simulink model "aerosonde_controlled"  (Simulink 7.7)
settings: Solver=ode3  StartTime=0.0  StopTime=200  FixedStep=20e-3  RelTol=1e-6
values from neighbouring files (symbols this model uses):
  aerosonde = aerosonde_data    [aerosonde_initialize.m]    (also in aerosonde_trimlin.m)
  chi_trim = 0    [aerosonde_initialize.m]
  eta_trim = -0.1    [aerosonde_initialize.m]
  euler_0 = [theta_trim; 0; 0]    [aerosonde_initialize.m]    (also in aerosonde_trimlin.m = xtrim(11:13))
  flap = 0    [aerosonde_initialize.m]
  fuel_0 = 2    [aerosonde_initialize.m]    (also in aerosonde_trimlin.m = xtrim(10))
  h_trim = 500    [aerosonde_initialize.m]
  ignition = 1    [aerosonde_initialize.m]
  Kari = 0.5    [aerosonde_initialize.m]
  Kd_Ye = 0.6    [aerosonde_initialize.m]
  Kd_Ze = -0.05    [aerosonde_initialize.m]
  Ki_phi = -0.1    [aerosonde_initialize.m]
  Ki_psi = 0.001    [aerosonde_initialize.m]
  Ki_theta = -0.8    [aerosonde_initialize.m]
  Ki_u = 0.15    [aerosonde_initialize.m]
  Ki_Ye = 0.0025    [aerosonde_initialize.m]
  Ki_Ze = -0.0001    [aerosonde_initialize.m]
  Kp_phi = -0.2    [aerosonde_initialize.m]
  Kp_psi = 0.7    [aerosonde_initialize.m]
  Kp_theta = -0.8    [aerosonde_initialize.m]
  Kp_u = 0.5    [aerosonde_initialize.m]
  Kp_Xe = 0.125    [aerosonde_initialize.m]
  Kp_Ye = 0.18    [aerosonde_initialize.m]
  Kp_Ze = -0.03    [aerosonde_initialize.m]
  Kphi_xi = -0.2    [aerosonde_initialize.m]
  Kq_eta = -0.28    [aerosonde_initialize.m]
  Kr_zeta = -0.25    [aerosonde_initialize.m]
  Ktheta_eta = -1    [aerosonde_initialize.m]
  latitude = 52.073105    [aerosonde_initialize.m]
  longitude = -000.616697    (= -0.616697)    [aerosonde_initialize.m]
  mixture = 13    [aerosonde_initialize.m]
  Omega_0 = 5000*pi/30    (= 523.598775598)    [aerosonde_initialize.m]    (also in aerosonde_trimlin.m = xtrim(14))
  position_0 = [0; 0; -h_trim]    [aerosonde_initialize.m]
  q_trim = 0    [aerosonde_initialize.m]
  rates_0 = [0; q_trim ; 0]    [aerosonde_initialize.m]    (also in aerosonde_trimlin.m = xtrim(7:9))
  tau_trim = 0.4    [aerosonde_initialize.m]
  theta_trim = 0    [aerosonde_initialize.m]
  Tr = 0.75    [aerosonde_initialize.m]
  Ue_VL = 25    [aerosonde_initialize.m]
  Ve_VL = 0    [aerosonde_initialize.m]
  velocity_0 = [23; 0; 0]    [aerosonde_initialize.m]    (also in aerosonde_trimlin.m = xtrim(1:3))
  We_VL = 0    [aerosonde_initialize.m]
  Xe0_VL = position_0(1)    [aerosonde_initialize.m]
  xi_trim = 0    [aerosonde_initialize.m]
  Ye0_VL = position_0(2)    [aerosonde_initialize.m]
  Ze0_VL = position_0(3)    [aerosonde_initialize.m]
  zeta_trim = 0    [aerosonde_initialize.m]
undefined symbols (not defined in the file or in its folder): Earth, F, m, MIL, rad, s, WGS84
libraries: aerolibasang x4, aerolibbdyn x3, aerolibfltsims x3, simulink_extras x3, aerolibwind2 x3, aerolibtransform2 x2, aerolibatmos2 x2, aerolibconvert2 x2, simulink x2, aerolibadyn x1, aerolib6dof2 x1, aerolibutil x1
(part 2 of 2)

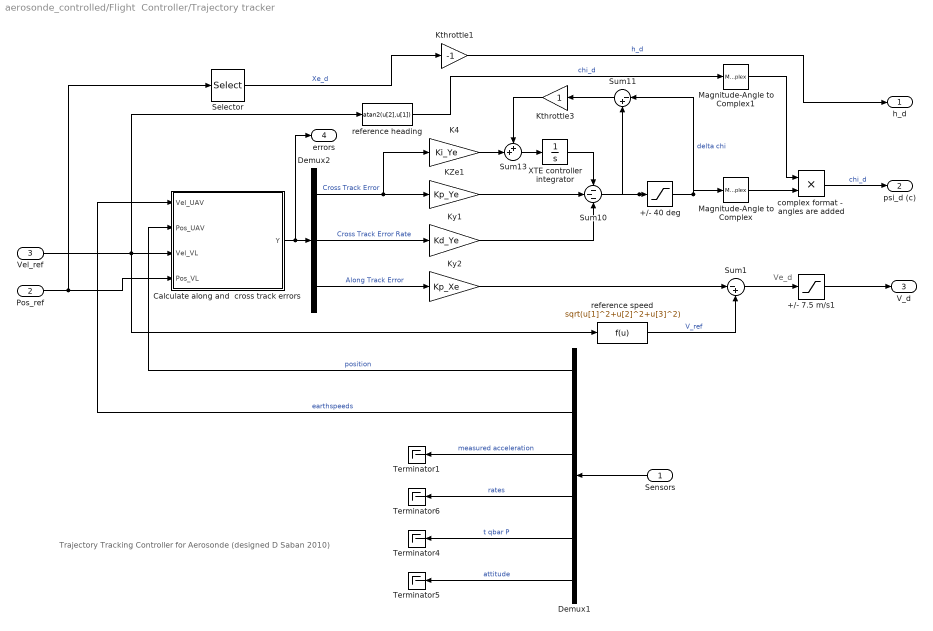
== system aerosonde_controlled/Flight  Controller/Trajectory tracker ==
  note: Ve_d
  note: Trajectory Tracking Controller
      | for Aerosonde
      | (designed D Saban 2010)
  Sensors : Inport  PortDimensions=18
  Pos_ref : Inport  Port=2
  Vel_ref : Inport  Port=3
  +/- 40 deg : Saturate  UpperLimit=+40.0*pi/180  LowerLimit=-40*pi/180  ZeroCross=off
  +/- 7.5 m/s1 : Saturate  UpperLimit=90  LowerLimit=18  ZeroCross=off
  Calculate along and  cross track errors : Stateflow chart  TreatAsAtomicUnit=on
  Demux1 : Demux  Outputs=[3 3 3 3 3 3]
  Demux2 : Demux  Outputs=3
  K4 : Gain  Gain=Ki_Ye
  KZe1 : Gain  Gain=Kp_Ye
  Kthrottle1 : Gain  Gain=-1
  Kthrottle3 : Gain
  Ky1 : Gain  Gain=Kd_Ye
  Ky2 : Gain  Gain=Kp_Xe
  Magnitude-Angle to Complex : MagnitudeAngleToComplex  Input=Angle  ConstantPart=1
  Magnitude-Angle to Complex1 : MagnitudeAngleToComplex  Input=Angle  ConstantPart=1
  Selector : Selector  InputPortWidth=3  IndexOptions=Index vector (dialog)  Indices=3  OutputSizes=1
  Sum1 : Sum  Inputs=|-+
  Sum10 : Sum  Inputs=---
  Sum11 : Sum  Inputs=|-+
  Sum13 : Sum  Inputs=++|
  Terminator{1,4..6} (4 alike) : Terminator
  XTE controller integrator : Integrator
  complex format -  angles are added : Product  RndMeth=Zero
  reference heading : Fcn  Expr=atan2(u[2],u[1])
  reference speed : Fcn  Expr=sqrt(u[1]^2+u[2]^2+u[3]^2)
  h_d : Outport
  psi_d (c) : Outport  Port=2
  V_d : Outport  Port=3
  errors : Outport  Port=4
  wires:
  KZe1/1 -> Sum10/2
  K4/1 -> Sum13/2
  Sum13/1 -> XTE controller integrator/1
  XTE controller integrator/1 -> Sum10/1
  Sum10/1 -> Sum11/2, +/- 40 deg/1
  Sum11/1 -> Kthrottle3/1
  Kthrottle3/1 -> Sum13/1
  Ky1/1 -> Sum10/3
  Demux2/1 -> KZe1/1, K4/1  "Cross Track Error"
  Calculate along and  cross track errors/1(Y) -> Demux2/1, errors/1
  Ky2/1 -> Sum1/1
  Pos_ref/1 -> Calculate along and  cross track errors/4(Pos_VL), Selector/1
  Vel_ref/1 -> Calculate along and  cross track errors/3(Vel_VL), reference speed/1, reference heading/1
  Demux2/3 -> Ky2/1  "Along Track Error"
  Demux2/2 -> Ky1/1  "Cross Track Error Rate"
  Demux1/2 -> Calculate along and  cross track errors/1(Vel_UAV)  "earthspeeds"
  Demux1/3 -> Terminator1/1  "measured acceleration"
  Sensors/1 -> Demux1/1
  Demux1/5 -> Terminator4/1  "t qbar P"
  Demux1/1 -> Calculate along and  cross track errors/2(Pos_UAV)  "position"
  Demux1/4 -> Terminator6/1  "rates"
  Demux1/6 -> Terminator5/1  "attitude"
  Selector/1 -> Kthrottle1/1  "Xe_d"
  Kthrottle1/1 -> h_d/1  "h_d"
  Sum1/1 -> +/- 7.5 m/s1/1
  reference speed/1 -> Sum1/2  "V_ref"
  +/- 7.5 m/s1/1 -> V_d/1
  complex format -  angles are added/1 -> psi_d (c)/1  "chi_d"
  +/- 40 deg/1 -> Sum11/1, Magnitude-Angle to Complex/1  "delta chi"
  reference heading/1 -> Magnitude-Angle to Complex1/1  "chi_d"
  Magnitude-Angle to Complex/1 -> complex format -  angles are added/2
  Magnitude-Angle to Complex1/1 -> complex format -  angles are added/1

== system aerosonde_controlled/FlightGear visualization/Flat Earth to LLA ==
  note: Flat Earth to LLA
  Xe : Inport
  altitude0 : Inport  Port=2
  Angle Conversion : aerolibconvert2/Angle Conversion  SystemSampleTime=-1  IU=deg  OU=rad
  Demux2 : Demux  Outputs=2
  Flat Earth to LLA : aerolibtransform2/Flat Earth to LLA  SystemSampleTime=-1  units=Metric (MKS)  ptype=Earth (WGS84)  F=1/298.257223563  R=6378137  LL0=[latitude longitude]  psi=0
  longitude l : Outport
  latitude mu : Outport  Port=2
  altitude h : Outport  Port=3
  wires:
  Flat Earth to LLA/1 -> Angle Conversion/1
  Demux2/1 -> latitude mu/1  "latitude"
  Demux2/2 -> longitude l/1
  Xe/1 -> Flat Earth to LLA/1
  altitude0/1 -> Flat Earth to LLA/2
  Flat Earth to LLA/2 -> altitude h/1  "altitude"
  Angle Conversion/1 -> Demux2/1

== system aerosonde_controlled/FlightGear visualization/phidot thetadot psidot ==
  pqr : Inport
  phi theta psi : Inport  Port=2
  Concatenate1 : Concatenate  NumInputs=3  Mode=Vector
  Concatenate2 : Concatenate  NumInputs=3  Mode=Vector
  SinCos : aerolibobsolete/SinCos  SystemSampleTime=-1
  keep angles  in range [-pi pi] : Trigonometry  Operator=atan2
  phidot : Fcn  Expr=u[1]+(u[2]*u[4]+u[3]*u[7])*(u[5]/u[8])
  psidot : Fcn  Expr=(u[2]*u[4]+u[3]*u[7])/u[8]
  thetadot : Fcn  Expr=u[2]*u[7]-u[3]*u[4]
  ptp_earth : Outport
  ptp_dot : Outport  Port=2
  wires:
  SinCos/2 -> Concatenate1/3, keep angles  in range [-pi pi]/2
  SinCos/1 -> Concatenate1/2, keep angles  in range [-pi pi]/1
  Concatenate2/1 -> ptp_dot/1
  phidot/1 -> Concatenate2/1
  thetadot/1 -> Concatenate2/2
  psidot/1 -> Concatenate2/3
  phi theta psi/1 -> SinCos/1
  pqr/1 -> Concatenate1/1
  Concatenate1/1 -> thetadot/1, phidot/1, psidot/1
  keep angles  in range [-pi pi]/1 -> ptp_earth/1

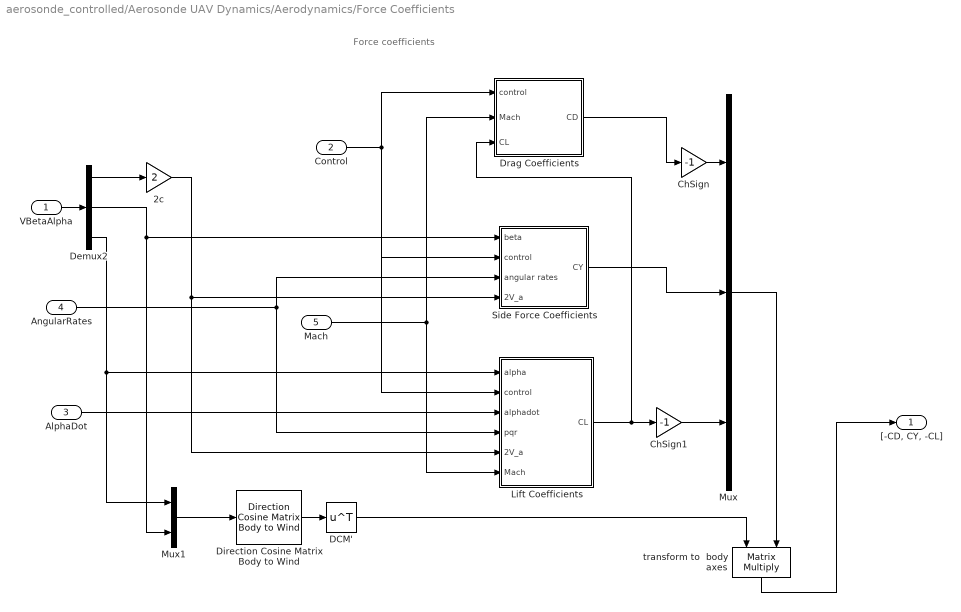
== system aerosonde_controlled/Aerosonde UAV Dynamics/Aerodynamics/Force Coefficients ==
  note: Force coefficients
  VBetaAlpha : Inport  PortDimensions=[3 1]
  Control : Inport  Port=2  PortDimensions=[4 1]
  AlphaDot : Inport  Port=3
  AngularRates : Inport  Port=4  PortDimensions=[3 1]
  Mach : Inport  Port=5  PortDimensions=1
  2c : Gain  Gain=2  SaturateOnIntegerOverflow=on  OutDataTypeStr=Inherit: Same as input  ParamDataTypeStr=Inherit: Same as input
  ChSign : Gain  Gain=-1  SaturateOnIntegerOverflow=on  OutDataTypeStr=Inherit: Same as input  ParamDataTypeStr=Inherit: Same as input
  ChSign1 : Gain  Gain=-1  SaturateOnIntegerOverflow=on  OutDataTypeStr=Inherit: Same as input  ParamDataTypeStr=Inherit: Same as input
  DCM' : Math  Operator=transpose  SaturateOnIntegerOverflow=on
  Demux2 : Demux  Outputs=3
  Direction Cosine Matrix Body to Wind : aerolibtransform2/Direction Cosine Matrix Body to Wind  SystemSampleTime=-1
  Drag Coefficients : Subsystem
  Lift Coefficients : Subsystem
  Mux : Mux  Inputs=3
  Mux1 : Mux  Inputs=2
  Side Force Coefficients : Subsystem
  transform to  body axes : Product  Inputs=**  Multiplication=Matrix(*)  SaturateOnIntegerOverflow=on  InputSameDT=on  OutDataTypeStr=Inherit: Same as first input
  "[-CD, CY, -CL]" : Outport
  wires:
  Mux1/1 -> Direction Cosine Matrix Body to Wind/1
  DCM'/1 -> transform to  body axes/1
  Mux/1 -> transform to  body axes/2
  Direction Cosine Matrix Body to Wind/1 -> DCM'/1
  transform to  body axes/1 -> "[-CD, CY, -CL]"/1
  Demux2/2 -> Mux1/2, Side Force Coefficients/1(beta)
  Demux2/1 -> 2c/1
  VBetaAlpha/1 -> Demux2/1
  ChSign1/1 -> Mux/3
  ChSign/1 -> Mux/1
  Side Force Coefficients/1(CY) -> Mux/2
  Drag Coefficients/1(CD) -> ChSign/1
  Lift Coefficients/1(CL) -> Drag Coefficients/3(CL), ChSign1/1
  Mach/1 -> Drag Coefficients/2(Mach), Lift Coefficients/6(Mach)
  AngularRates/1 -> Side Force Coefficients/3(angular rates), Lift Coefficients/4(pqr)
  AlphaDot/1 -> Lift Coefficients/3(alphadot)
  Control/1 -> Lift Coefficients/2(control), Side Force Coefficients/2(control), Drag Coefficients/1(control)
  Demux2/3 -> Lift Coefficients/1(alpha), Mux1/1
  2c/1 -> Side Force Coefficients/4(2V_a), Lift Coefficients/5(2V_a)

== system aerosonde_controlled/Aerosonde UAV Dynamics/Aerodynamics/Moment Coefficients ==
  note: Moment coefficients
  VBetaAlpha : Inport  PortDimensions=[3 1]
  Control : Inport  Port=2  PortDimensions=[4 1]
  AlphaDot : Inport  Port=3
  AngularRates : Inport  Port=4  PortDimensions=[3 1]
  Mach : Inport  Port=5  PortDimensions=1
  2c : Gain  Gain=2  SaturateOnIntegerOverflow=on  OutDataTypeStr=Inherit: Same as input  ParamDataTypeStr=Inherit: Same as input
  Demux1 : Demux  Outputs=3
  Mux : Mux  Inputs=3
  Pitch Moment Coefficients : Subsystem
  Roll Moment Coefficients : Subsystem
  Yaw Moment Coefficients : Subsystem
  "[-Cl, Cm, -Cn]" : Outport
  wires:
  Demux1/2 -> Yaw Moment Coefficients/1(beta), Roll Moment Coefficients/1(beta)
  Demux1/3 -> Pitch Moment Coefficients/1(alpha)
  Mach/1 -> Pitch Moment Coefficients/6(Mach)
  Yaw Moment Coefficients/1(Cn) -> Mux/3
  VBetaAlpha/1 -> Demux1/1
  2c/1 -> Pitch Moment Coefficients/5(2V_a), Yaw Moment Coefficients/4(2V_a), Roll Moment Coefficients/4(2V)
  Demux1/1 -> 2c/1
  Control/1 -> Roll Moment Coefficients/2(control), Yaw Moment Coefficients/2(control), Pitch Moment Coefficients/2(control)
  AlphaDot/1 -> Pitch Moment Coefficients/3(alphadot)
  AngularRates/1 -> Roll Moment Coefficients/3(angular rates), Yaw Moment Coefficients/3(angular rates), Pitch Moment Coefficients/4(pqr)
  Mux/1 -> "[-Cl, Cm, -Cn]"/1
  Pitch Moment Coefficients/1(Cm) -> Mux/2
  Roll Moment Coefficients/1(Cl) -> Mux/1

== system aerosonde_controlled/Aerosonde UAV Dynamics/Aerodynamics/Wind-axes Velocities ==
  VelB : Inport
  WindB : Inport  Port=2
  a : Inport  Port=3
  rho : Inport  Port=4
  VelBdot : Inport  Port=5
  Calculate  alphadot : Subsystem
  Derivative : Derivative
  Dynamic Pressure : aerolibasang/Dynamic Pressure  SystemSampleTime=-1
  "Incidence, Sideslip, & Airspeed" : aerolibasang/Incidence, Sideslip, & Airspeed  SystemSampleTime=-1
  Mach Number : aerolibasang/Mach Number  SystemSampleTime=-1
  Mux1 : Mux  Inputs=3
  Sum1 : Sum  Inputs=|+-  SaturateOnIntegerOverflow=on  InputSameDT=on  OutDataTypeStr=Inherit: Same as first input
  Sum2 : Sum  Inputs=-+|  SaturateOnIntegerOverflow=on  InputSameDT=on  OutDataTypeStr=Inherit: Same as first input
  VBetaAlpha : Outport
  Mach : Outport  Port=2
  qbar (pdyn) : Outport  Port=3
  alphadot : Outport  Port=4
  wires:
  Derivative/1 -> Sum2/1
  Sum2/1 -> Calculate  alphadot/1("[Udot Vdot Wdot]")
  VelBdot/1 -> Sum2/2
  Calculate  alphadot/1(alphadot) -> alphadot/1
  "Incidence, Sideslip, & Airspeed"/2 -> Mux1/2
  "Incidence, Sideslip, & Airspeed"/1 -> Mux1/3
  Dynamic Pressure/1 -> qbar (pdyn)/1
  rho/1 -> Dynamic Pressure/2
  a/1 -> Mach Number/2
  Mach Number/1 -> Mach/1
  WindB/1 -> Derivative/1, Sum1/2
  VelB/1 -> Sum1/1
  Mux1/1 -> VBetaAlpha/1
  "Incidence, Sideslip, & Airspeed"/3 -> Mux1/1
  Sum1/1 -> Calculate  alphadot/2("[U V W]"), Dynamic Pressure/1, Mach Number/1, "Incidence, Sideslip, & Airspeed"/1

== system aerosonde_controlled/Aerosonde UAV Dynamics/Propulsion System/Fixed-pitch Propeller ==
  note: Fixed-pitch
      | Propeller
  Airspeed : Inport  OutDataTypeStr=double  PortDimensions=1
  rho : Inport  Port=2  OutDataTypeStr=double  PortDimensions=1
  Omega : Inport  Port=3  OutDataTypeStr=double  PortDimensions=1
  4 R^4 / pi^2 : Gain  Gain=4*Rprop^4/pi^2  SaturateOnIntegerOverflow=on  OutDataTypeStr=Inherit: Same as input  ParamDataTypeStr=Inherit: Same as input
  4 R^5/ pi^3 : Gain  Gain=-4*Rprop^5/pi^3  SaturateOnIntegerOverflow=on  OutDataTypeStr=Inherit: Same as input  ParamDataTypeStr=Inherit: Same as input
  Coeff of Power : Lookup  InputValues=J  Table=CP  SaturateOnIntegerOverflow=on
  Coefficient  of Thrust : Lookup  InputValues=J  Table=CT  SaturateOnIntegerOverflow=on
  Omega^2 : Math  Operator=square  SaturateOnIntegerOverflow=on
  Va/Omega : Product  Inputs=*/  SaturateOnIntegerOverflow=on  InputSameDT=on  OutDataTypeStr=Inherit: Same as first input
  pi/R : Gain  Gain=pi/Rprop  SaturateOnIntegerOverflow=on  OutDataTypeStr=Inherit: Same as input  ParamDataTypeStr=Inherit: Same as input
  "rho Omega^2 " : Product  SaturateOnIntegerOverflow=on  InputSameDT=on  OutDataTypeStr=Inherit: Same as first input
  rho Omega^2 C_P : Product  SaturateOnIntegerOverflow=on  InputSameDT=on  OutDataTypeStr=Inherit: Same as first input
  rho Omega^2 C_T : Product  SaturateOnIntegerOverflow=on  InputSameDT=on  OutDataTypeStr=Inherit: Same as first input
  Fprop : Outport
  Mprop : Outport  Port=2
  wires:
  "rho Omega^2 "/1 -> rho Omega^2 C_P/2, rho Omega^2 C_T/2
  Omega^2/1 -> "rho Omega^2 "/1
  rho/1 -> "rho Omega^2 "/2
  4 R^5/ pi^3/1 -> Mprop/1  "torque"
  4 R^4 / pi^2/1 -> Fprop/1  "thrust"
  Airspeed/1 -> Va/Omega/1
  pi/R/1 -> Coeff of Power/1, Coefficient  of Thrust/1  "advance ratio"
  rho Omega^2 C_P/1 -> 4 R^5/ pi^3/1
  rho Omega^2 C_T/1 -> 4 R^4 / pi^2/1
  Coefficient  of Thrust/1 -> rho Omega^2 C_T/1
  Va/Omega/1 -> pi/R/1
  Omega/1 -> Va/Omega/2, Omega^2/1
  Coeff of Power/1 -> rho Omega^2 C_P/1

== system aerosonde_controlled/Aerosonde UAV Dynamics/Propulsion System/Piston Engine ==
  note: Compute MAP from
      | throttle area fraction
  note: Engine parameter
      | look-up tables
  Thr : Inport  OutDataTypeStr=double  PortDimensions=1
  Mix : Inport  Port=2  OutDataTypeStr=double  PortDimensions=1
  Omega : Inport  Port=3  OutDataTypeStr=double  PortDimensions=1
  P_atm : Inport  Port=4  OutDataTypeStr=double  PortDimensions=1
  T : Inport  Port=5  OutDataTypeStr=double  PortDimensions=1
  Altitude correction  for  Power : Subsystem
  Engine torque : Product  Inputs=*/  SaturateOnIntegerOverflow=on  InputSameDT=on  OutDataTypeStr=Inherit: Same as first input
  Fuel flow LUT : Lookup2D  RowIndex=RPM  ColumnIndex=MAP  Table=fflow  SaturateOnIntegerOverflow=on  InputSameDT=on
  Get air flow : Product  SaturateOnIntegerOverflow=on  InputSameDT=on  OutDataTypeStr=Inherit: Same as first input
  Intake : Subsystem
  Power LUT : Lookup2D  RowIndex=RPM  ColumnIndex=MAP  Table=Power  SaturateOnIntegerOverflow=on  InputSameDT=on
  Power at altitude : Product  SaturateOnIntegerOverflow=on  InputSameDT=on  OutDataTypeStr=Inherit: Same as first input
  g/hr 2 kg/s : Gain  Gain=1/1000/3600  SaturateOnIntegerOverflow=on  OutDataTypeStr=Inherit: Same as input  ParamDataTypeStr=Inherit: Same as input
  rad/s 2 RPM : Gain  Gain=30/pi  SaturateOnIntegerOverflow=on  OutDataTypeStr=Inherit: Same as input  ParamDataTypeStr=Inherit: Same as input
  AirFlow : Outport
  FuelFlow : Outport  Port=2
  Torque : Outport  Port=3
  wires:
  Get air flow/1 -> AirFlow/1
  Mix/1 -> Get air flow/2
  Intake/1(MAP) -> Power LUT/2, Fuel flow LUT/2
  g/hr 2 kg/s/1 -> Get air flow/1, FuelFlow/1
  Omega/1 -> rad/s 2 RPM/1, Engine torque/2
  rad/s 2 RPM/1 -> Fuel flow LUT/1, Power LUT/1
  T/1 -> Altitude correction  for  Power/1(T)
  Power LUT/1 -> Power at altitude/1
  Altitude correction  for  Power/1(Power correction) -> Power at altitude/2
  Power at altitude/1 -> Engine torque/1
  Fuel flow LUT/1 -> g/hr 2 kg/s/1
  Engine torque/1 -> Torque/1
  Thr/1 -> Intake/1(Thr)
  P_atm/1 -> Intake/2(P_atm)

== system aerosonde_controlled/Flight  Controller/Autopilot/speed 2 angle (c) ==
  speed : Inport
  Demux : Demux  Outputs=3
  Real-Imag to Complex : RealImagToComplex
  Terminator2 : Terminator
  Re Im : Outport
  wires:
  speed/1 -> Demux/1
  Real-Imag to Complex/1 -> Re Im/1
  Demux/3 -> Terminator2/1
  Demux/2 -> Real-Imag to Complex/2
  Demux/1 -> Real-Imag to Complex/1

== system aerosonde_controlled/Aerosonde UAV Dynamics/Aerodynamics/Force Coefficients/Drag Coefficients ==
  note: Drag coefficient
  control : Inport
  Mach : Inport  Port=2
  CL : Inport  Port=3  PortDimensions=1
  (CL-CL0)^2/(pi e AR) : Gain  Gain=1/as.pieaR  Multiplication=Matrix(K*u)  SaturateOnIntegerOverflow=on  OutDataTypeStr=Inherit: Same as input  ParamDataTypeStr=Inherit: Same as input
  Abs4 : Abs  SaturateOnIntegerOverflow=on
  CDM : Gain  Gain=as.CDM  SaturateOnIntegerOverflow=on  OutDataTypeStr=Inherit: Same as input  ParamDataTypeStr=Inherit: Same as input
  CDdf : Gain  Gain=[as.CDdf, as.CDde, as.CDda, as.CDdr]  Multiplication=Matrix(K*u)  SaturateOnIntegerOverflow=on  OutDataTypeStr=Inherit: Same as input  ParamDataTypeStr=Inherit: Same as input
  CL min drag : Constant  Value=as.CLmind
  CL^2 : Math  Operator=square  SaturateOnIntegerOverflow=on
  Constant terms : Constant  Value=as.CD0
  Sum : Sum  Inputs=|+-  SaturateOnIntegerOverflow=on  InputSameDT=on  OutDataTypeStr=Inherit: Same as first input
  Sum1 : Sum  Inputs=++++  SaturateOnIntegerOverflow=on  InputSameDT=on  OutDataTypeStr=Inherit: Same as first input
  CD : Outport
  wires:
  (CL-CL0)^2/(pi e AR)/1 -> Sum1/4
  CL min drag/1 -> Sum/2
  CL/1 -> Sum/1
  Sum/1 -> CL^2/1
  CL^2/1 -> (CL-CL0)^2/(pi e AR)/1
  Sum1/1 -> CD/1  "CD"
  Mach/1 -> CDM/1
  control/1 -> Abs4/1
  Abs4/1 -> CDdf/1
  CDM/1 -> Sum1/3
  CDdf/1 -> Sum1/2
  Constant terms/1 -> Sum1/1

== system aerosonde_controlled/Aerosonde UAV Dynamics/Aerodynamics/Force Coefficients/Lift Coefficients ==
  note: Lift Coefficients
  alpha : Inport
  control : Inport  Port=2
  alphadot : Inport  Port=3
  pqr : Inport  Port=4
  2V_a : Inport  Port=5
  Mach : Inport  Port=6
  CL*c/(2V_a) : Product  Inputs=*/  SaturateOnIntegerOverflow=on  InputSameDT=on  OutDataTypeStr=Inherit: Same as first input
  CL0 : Constant  Value=as.CL0
  CLM : Gain  Gain=as.CLM  SaturateOnIntegerOverflow=on  OutDataTypeStr=Inherit: Same as input  ParamDataTypeStr=Inherit: Same as input
  CLalpha : Gain  Gain=as.CLalpha  SaturateOnIntegerOverflow=on  OutDataTypeStr=Inherit: Same as input  ParamDataTypeStr=Inherit: Same as input
  CLalphadot : Gain  Gain=as.CLalphadot  Multiplication=Matrix(K*u)  SaturateOnIntegerOverflow=on  OutDataTypeStr=Inherit: Same as input  ParamDataTypeStr=Inherit: Same as input
  CLq : Gain  Gain=[0, as.CLq, 0]  Multiplication=Matrix(K*u)  SaturateOnIntegerOverflow=on  OutDataTypeStr=Inherit: Same as input  ParamDataTypeStr=Inherit: Same as input
  Sum : Sum  SaturateOnIntegerOverflow=on  InputSameDT=on  OutDataTypeStr=Inherit: Same as first input
  Sum2 : Sum  Inputs=+++++  SaturateOnIntegerOverflow=on  InputSameDT=on  OutDataTypeStr=Inherit: Same as first input
  "[CLdf, CLde, 0, 0]" : Gain  Gain=[as.CLdf, as.CLde, 0, 0]  Multiplication=Matrix(K*u)  SaturateOnIntegerOverflow=on  OutDataTypeStr=Inherit: Same as input  ParamDataTypeStr=Inherit: Same as input
  c : Gain  Gain=as.c  SaturateOnIntegerOverflow=on  OutDataTypeStr=Inherit: Same as input  ParamDataTypeStr=Inherit: Same as input
  CL : Outport
  wires:
  alphadot/1 -> CLalphadot/1
  alpha/1 -> CLalpha/1
  Mach/1 -> CLM/1
  2V_a/1 -> CL*c/(2V_a)/2
  pqr/1 -> CLq/1
  control/1 -> "[CLdf, CLde, 0, 0]"/1
  c/1 -> CL*c/(2V_a)/1
  CL*c/(2V_a)/1 -> Sum2/4
  CLM/1 -> Sum2/5
  Sum2/1 -> CL/1  "CL"
  "[CLdf, CLde, 0, 0]"/1 -> Sum2/3
  CLalpha/1 -> Sum2/2
  CL0/1 -> Sum2/1
  Sum/1 -> c/1
  CLalphadot/1 -> Sum/1
  CLq/1 -> Sum/2

== system aerosonde_controlled/Aerosonde UAV Dynamics/Aerodynamics/Force Coefficients/Side Force Coefficients ==
  note: Side force coefficients
  beta : Inport
  control : Inport  Port=2
  angular rates : Inport  Port=3
  2V_a : Inport  Port=4
  CY*b/(2V_a) : Product  Inputs=*/  SaturateOnIntegerOverflow=on  InputSameDT=on  OutDataTypeStr=Inherit: Same as first input
  CYbeta : Gain  Gain=as.CYbeta  SaturateOnIntegerOverflow=on  OutDataTypeStr=Inherit: Same as input  ParamDataTypeStr=Inherit: Same as input
  Sum3 : Sum  Inputs=+++  SaturateOnIntegerOverflow=on  InputSameDT=on  OutDataTypeStr=Inherit: Same as first input
  Wing span1 : Gain  Gain=as.b  SaturateOnIntegerOverflow=on  OutDataTypeStr=Inherit: Same as input  ParamDataTypeStr=Inherit: Same as input
  "[0, 0, CYda, CYdr]" : Gain  Gain=[0, 0, as.CYda, as.CYdr]  Multiplication=Matrix(K*u)  SaturateOnIntegerOverflow=on  OutDataTypeStr=Inherit: Same as input  ParamDataTypeStr=Inherit: Same as input
  "[CYp, 0, CYr]" : Gain  Gain=[as.CYp, 0, as.CYr]  Multiplication=Matrix(K*u)  SaturateOnIntegerOverflow=on  OutDataTypeStr=Inherit: Same as input  ParamDataTypeStr=Inherit: Same as input
  CY : Outport
  wires:
  beta/1 -> CYbeta/1
  2V_a/1 -> CY*b/(2V_a)/2
  angular rates/1 -> "[CYp, 0, CYr]"/1
  control/1 -> "[0, 0, CYda, CYdr]"/1
  Wing span1/1 -> CY*b/(2V_a)/1
  Sum3/1 -> CY/1  "CY"
  CY*b/(2V_a)/1 -> Sum3/3
  "[0, 0, CYda, CYdr]"/1 -> Sum3/2
  CYbeta/1 -> Sum3/1
  "[CYp, 0, CYr]"/1 -> Wing span1/1

== system aerosonde_controlled/Aerosonde UAV Dynamics/Aerodynamics/Moment Coefficients/Pitch Moment Coefficients ==
  alpha : Inport
  control : Inport  Port=2
  alphadot : Inport  Port=3
  pqr : Inport  Port=4
  2V_a : Inport  Port=5
  Mach : Inport  Port=6
  CMalpha : Gain  Gain=as.Cmalpha  SaturateOnIntegerOverflow=on  OutDataTypeStr=Inherit: Same as input  ParamDataTypeStr=Inherit: Same as input
  Cm*c/(2V_a) : Product  Inputs=*/  SaturateOnIntegerOverflow=on  InputSameDT=on  OutDataTypeStr=Inherit: Same as first input
  Cm0 : Constant  Value=as.Cm0
  CmM : Gain  Gain=as.CmM  SaturateOnIntegerOverflow=on  OutDataTypeStr=Inherit: Same as input  ParamDataTypeStr=Inherit: Same as input
  Cmalphadot : Gain  Gain=as.Cmalphadot  Multiplication=Matrix(K*u)  SaturateOnIntegerOverflow=on  OutDataTypeStr=Inherit: Same as input  ParamDataTypeStr=Inherit: Same as input
  Cmq : Gain  Gain=[0, as.Cmq, 0]  Multiplication=Matrix(K*u)  SaturateOnIntegerOverflow=on  OutDataTypeStr=Inherit: Same as input  ParamDataTypeStr=Inherit: Same as input
  Sum : Sum  SaturateOnIntegerOverflow=on  InputSameDT=on  OutDataTypeStr=Inherit: Same as first input
  Sum2 : Sum  Inputs=+++++  SaturateOnIntegerOverflow=on  InputSameDT=on  OutDataTypeStr=Inherit: Same as first input
  "[Cmdf, Cmde, 0, 0]" : Gain  Gain=[as.Cmdf, as.Cmde, 0, 0]  Multiplication=Matrix(K*u)  SaturateOnIntegerOverflow=on  OutDataTypeStr=Inherit: Same as input  ParamDataTypeStr=Inherit: Same as input
  c : Gain  Gain=as.c  SaturateOnIntegerOverflow=on  OutDataTypeStr=Inherit: Same as input  ParamDataTypeStr=Inherit: Same as input
  Cm : Outport
  wires:
  Cmq/1 -> Sum/2
  Cmalphadot/1 -> Sum/1
  Sum/1 -> c/1
  Cm0/1 -> Sum2/1
  CMalpha/1 -> Sum2/2
  "[Cmdf, Cmde, 0, 0]"/1 -> Sum2/3
  Sum2/1 -> Cm/1  "Cm"
  CmM/1 -> Sum2/5
  Cm*c/(2V_a)/1 -> Sum2/4
  c/1 -> Cm*c/(2V_a)/1
  control/1 -> "[Cmdf, Cmde, 0, 0]"/1
  pqr/1 -> Cmq/1
  2V_a/1 -> Cm*c/(2V_a)/2
  Mach/1 -> CmM/1
  alpha/1 -> CMalpha/1
  alphadot/1 -> Cmalphadot/1

== system aerosonde_controlled/Aerosonde UAV Dynamics/Aerodynamics/Moment Coefficients/Roll Moment Coefficients ==
  note: Roll moment coefficient
  beta : Inport
  control : Inport  Port=2
  angular rates : Inport  Port=3
  2V : Inport  Port=4
  CY*b/(2V) : Product  Inputs=*/  SaturateOnIntegerOverflow=on  InputSameDT=on  OutDataTypeStr=Inherit: Same as first input
  Clbeta : Gain  Gain=as.Clbeta  SaturateOnIntegerOverflow=on  OutDataTypeStr=Inherit: Same as input  ParamDataTypeStr=Inherit: Same as input
  Sum3 : Sum  Inputs=+++  SaturateOnIntegerOverflow=on  InputSameDT=on  OutDataTypeStr=Inherit: Same as first input
  Wing span : Gain  Gain=as.b  SaturateOnIntegerOverflow=on  OutDataTypeStr=Inherit: Same as input  ParamDataTypeStr=Inherit: Same as input
  "[0, 0, Clda, Cldr]" : Gain  Gain=[0, 0, as.Clda, as.Cldr]  Multiplication=Matrix(K*u)  SaturateOnIntegerOverflow=on  OutDataTypeStr=Inherit: Same as input  ParamDataTypeStr=Inherit: Same as input
  "[Clp, 0, Clr]" : Gain  Gain=[as.Clp, 0, as.Clr]  Multiplication=Matrix(K*u)  SaturateOnIntegerOverflow=on  OutDataTypeStr=Inherit: Same as input  ParamDataTypeStr=Inherit: Same as input
  Cl : Outport
  wires:
  "[Clp, 0, Clr]"/1 -> Wing span/1
  Clbeta/1 -> Sum3/1
  "[0, 0, Clda, Cldr]"/1 -> Sum3/2
  CY*b/(2V)/1 -> Sum3/3
  Sum3/1 -> Cl/1  "Cl"
  Wing span/1 -> CY*b/(2V)/1
  control/1 -> "[0, 0, Clda, Cldr]"/1
  angular rates/1 -> "[Clp, 0, Clr]"/1
  2V/1 -> CY*b/(2V)/2
  beta/1 -> Clbeta/1

== system aerosonde_controlled/Aerosonde UAV Dynamics/Aerodynamics/Moment Coefficients/Yaw Moment Coefficients ==
  note: Yaw moment coefficient
  beta : Inport
  control : Inport  Port=2
  angular rates : Inport  Port=3
  2V_a : Inport  Port=4
  Cn*b/(2V_a) : Product  Inputs=*/  SaturateOnIntegerOverflow=on  InputSameDT=on  OutDataTypeStr=Inherit: Same as first input
  Cnbeta : Gain  Gain=as.Cnbeta  SaturateOnIntegerOverflow=on  OutDataTypeStr=Inherit: Same as input  ParamDataTypeStr=Inherit: Same as input
  Sum3 : Sum  Inputs=+++  SaturateOnIntegerOverflow=on  InputSameDT=on  OutDataTypeStr=Inherit: Same as first input
  Wing span : Gain  Gain=as.b  SaturateOnIntegerOverflow=on  OutDataTypeStr=Inherit: Same as input  ParamDataTypeStr=Inherit: Same as input
  "[0, 0, Cnda, Cndr]" : Gain  Gain=[0, 0, as.Cnda, as.Cndr]  Multiplication=Matrix(K*u)  SaturateOnIntegerOverflow=on  OutDataTypeStr=Inherit: Same as input  ParamDataTypeStr=Inherit: Same as input
  "[Cnp, 0, Cnr]" : Gain  Gain=[as.Cnp, 0, as.Cnr]  Multiplication=Matrix(K*u)  SaturateOnIntegerOverflow=on  OutDataTypeStr=Inherit: Same as input  ParamDataTypeStr=Inherit: Same as input
  Cn : Outport
  wires:
  beta/1 -> Cnbeta/1
  2V_a/1 -> Cn*b/(2V_a)/2
  angular rates/1 -> "[Cnp, 0, Cnr]"/1
  control/1 -> "[0, 0, Cnda, Cndr]"/1
  Wing span/1 -> Cn*b/(2V_a)/1
  Sum3/1 -> Cn/1  "Cn"
  Cn*b/(2V_a)/1 -> Sum3/3
  "[0, 0, Cnda, Cndr]"/1 -> Sum3/2
  Cnbeta/1 -> Sum3/1
  "[Cnp, 0, Cnr]"/1 -> Wing span/1

== system aerosonde_controlled/Aerosonde UAV Dynamics/Aerodynamics/Wind-axes Velocities/Calculate  alphadot ==
  note: Calculate alphadot
  note: W
  "[Udot Vdot Wdot]" : Inport
  "[U V W]" : Inport  Port=2
  Demux : Demux  Outputs=3
  Demux1 : Demux  Outputs=3
  Math Function : Math  Operator=square  SaturateOnIntegerOverflow=on
  Math Function1 : Math  Operator=square  SaturateOnIntegerOverflow=on
  Product : Product  RndMeth=Zero
  Product1 : Product  RndMeth=Zero
  Product2 : Product  Inputs=*/  RndMeth=Zero
  Sum : Sum  Inputs=-|+
  Sum1 : Sum  Inputs=+|+
  Terminator : Terminator
  Terminator1 : Terminator
  alphadot : Outport
  wires:
  Product2/1 -> alphadot/1  "alphadot"
  "[Udot Vdot Wdot]"/1 -> Demux/1
  "[U V W]"/1 -> Demux1/1
  Demux1/2 -> Terminator1/1
  Sum/1 -> Product2/1
  Product/1 -> Sum/2  "U Wdot"
  Product1/1 -> Sum/1  "W Udot"
  Sum1/1 -> Product2/2  "U^2 + W^2"
  Math Function1/1 -> Sum1/2
  Math Function/1 -> Sum1/1
  Demux1/3 -> Math Function1/1, Product1/2
  Demux1/1 -> Math Function/1, Product/2  "U"
  Demux/2 -> Terminator/1
  Demux/3 -> Product/1  "Wdot"
  Demux/1 -> Product1/1  "Udot"

== system aerosonde_controlled/Aerosonde UAV Dynamics/Propulsion System/Piston Engine/Altitude correction  for  Power ==
  note: Altitude correction for Power
  T : Inport
  Math Function : Math  Operator=sqrt  SaturateOnIntegerOverflow=on
  Product of Elements : Product  Inputs=/
  "Sea-level temperature " : Gain  Gain=TSL  SaturateOnIntegerOverflow=on  OutDataTypeStr=Inherit: Same as input  ParamDataTypeStr=Inherit: Same as input
  Power correction : Outport
  wires:
  T/1 -> Product of Elements/1
  Math Function/1 -> Power correction/1
  "Sea-level temperature "/1 -> Math Function/1
  Product of Elements/1 -> "Sea-level temperature "/1

== system aerosonde_controlled/Aerosonde UAV Dynamics/Propulsion System/Piston Engine/Intake ==
  Thr : Inport  OutDataTypeStr=double  PortDimensions=1
  P_atm : Inport  Port=2  OutDataTypeStr=double  PortDimensions=1
  Get MAP : Product  SaturateOnIntegerOverflow=on  InputSameDT=on  OutDataTypeStr=Inherit: Same as first input
  MAP min : Constant  Value=as.MAPmin
  Saturation : Saturate  UpperLimit=inf  LowerLimit=as.MAPmin
  Sum : Sum  Inputs=|+-  SaturateOnIntegerOverflow=on  InputSameDT=on  OutDataTypeStr=Inherit: Same as first input
  Sum1 : Sum  Inputs=|++  SaturateOnIntegerOverflow=on  InputSameDT=on  OutDataTypeStr=Inherit: Same as first input
  kPa : Gain  Gain=1/1000  SaturateOnIntegerOverflow=on  OutDataTypeStr=Inherit: Same as input  ParamDataTypeStr=Inherit: Same as input
  MAP : Outport
  wires:
  Saturation/1 -> MAP/1
  P_atm/1 -> kPa/1
  Thr/1 -> Get MAP/1
  MAP min/1 -> Sum/2, Sum1/2
  kPa/1 -> Sum/1
  Sum/1 -> Get MAP/2
  Get MAP/1 -> Sum1/1
  Sum1/1 -> Saturation/1

== matlab function Flight Controller/Trajectory tracker/Calculate along and cross track errors ==
  data: Vel_UAV input double; Pos_UAV input double; Vel_VL input double; Pos_VL input double; Y output double
function Y = track(Vel_UAV,Pos_UAV,Vel_VL,Pos_VL)

xVL = Pos_VL(1);
yVL = Pos_VL(2);
zVL = Pos_VL(3);

xUAV = Pos_UAV(1);
yUAV = Pos_UAV(2);
zUAV = Pos_UAV(3);

ChiVL = atan2(Vel_VL(2),Vel_VL(1));


% Distance between VL and UAV:
d_NED = [xUAV-xVL; yUAV-yVL; zUAV-zVL];

% Relative velocity between VL and UAV:
dV_NED = Vel_UAV - Vel_VL;

% Rotation matrix from NED to unD:
R = [cos(ChiVL) -sin(ChiVL) 0;
     sin(ChiVL)  cos(ChiVL) 0;
            0           0   1];

        
%----------------------------------------

d_unD = inv(R)*d_NED;
dV_unD = inv(R)*dV_NED;

ATD = d_unD(1);
OTD = d_unD(2);

dOTD = dV_unD(2);

%----------------------------------------

Y = [OTD; dOTD; ATD];
